simulink model "distributedPipelining"  (R2024a)
settings: Solver=FixedStepDiscrete  StartTime=0.0  StopTime=20/100e6  RelTol=1e-3
settings Model: DataTypeOverride=Off  Creator=cotti  LastModifiedBy=cotti
settings OptimizationCC: BlockReduction=off  ConditionallyExecuteInputs=off  DefaultParameterBehavior=Inlined  InheritOutputTypeSmallerThanSingle=on
settings DebuggingCC: AlgebraicLoopMsg=error  SingleTaskRateTransMsg=error  UnconnectedInputMsg=warning  UnconnectedOutputMsg=warning  UnconnectedLineMsg=warning
settings HardwareCC: ProdBitPerPointer=32  ProdBitPerSizeT=32  ProdBitPerPtrDiffT=32  ProdLargestAtomicFloat=None  ProdIntDivRoundTo=Undefined  ProdEndianess=Unspecified  ProdWordSize=32  ProdHWDeviceType=ASIC/FPGA->ASIC/FPGA  TargetBitPerLong=64  TargetBitPerPointer=64  TargetBitPerSizeT=64  TargetBitPerPtrDiffT=64  TargetLongLongMode=on  TargetIntDivRoundTo=Zero  TargetEndianess=LittleEndian  TargetWordSize=64  TargetHWDeviceType=Custom Processor->MATLAB Host Computer  ProdEqTarget=off

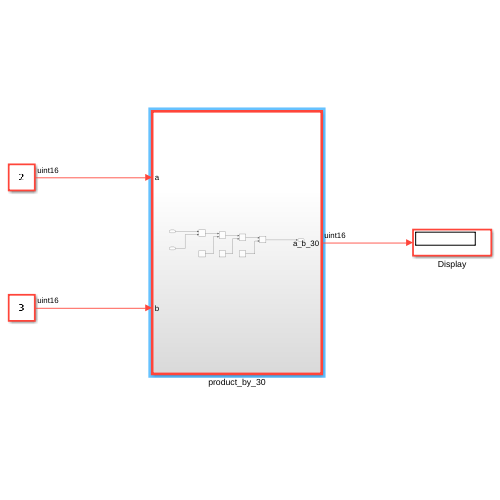
[thumbnail: Simulink's stored preview of the top-level diagram]
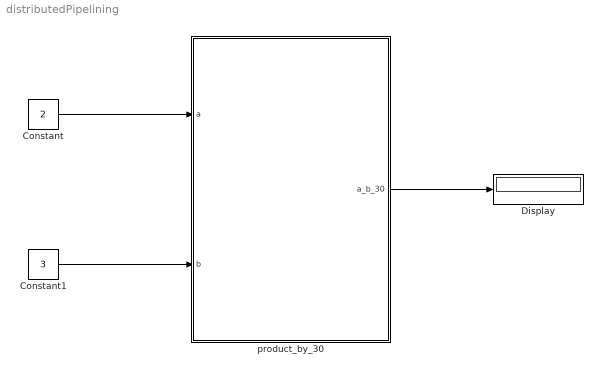
== system distributedPipelining ==
  Constant : Constant  Value=2  OutDataTypeStr=uint16  SampleTime=1/100e6
  Constant1 : Constant  Value=3  OutDataTypeStr=uint16  SampleTime=1/100e6
  Display : Display
  product_by_30 : Subsystem  TreatAsAtomicUnit=on
  wires:
  Constant/1 -> product_by_30/1(a)
  Constant1/1 -> product_by_30/2(b)
  product_by_30/1(a_b_30) -> Display/1

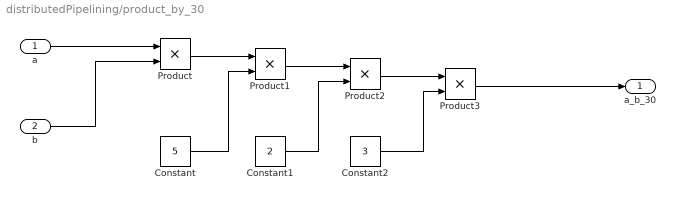
== system distributedPipelining/product_by_30 ==
  a : Inport
  b : Inport  Port=2
  Constant : Constant  Value=5  OutDataTypeStr=uint8  SampleTime=-1
  Constant1 : Constant  Value=2  OutDataTypeStr=uint8  SampleTime=-1
  Constant2 : Constant  Value=3  OutDataTypeStr=uint8  SampleTime=-1
  Product{,1..3} (4 alike) : Product  OutDataTypeStr=uint16
  a_b_30 : Outport
  wires:
  b/1 -> Product/2
  a/1 -> Product/1
  Constant/1 -> Product1/2
  Product1/1 -> Product2/1
  Constant1/1 -> Product2/2
  Product/1 -> Product1/1
  Product2/1 -> Product3/1
  Constant2/1 -> Product3/2
  Product3/1 -> a_b_30/1
